simulink model "DiscretePiController"  (R2023a)
settings: Solver=VariableStepAuto  StartTime=0.0  StopTime=10.0  RelTol=1e-3
model workspace (MAT data in the model file):
  Ts = 0.1
  ki = 1
  kp = 0.2
settings Model: Creator=MY PC  LastModifiedBy=MY PC

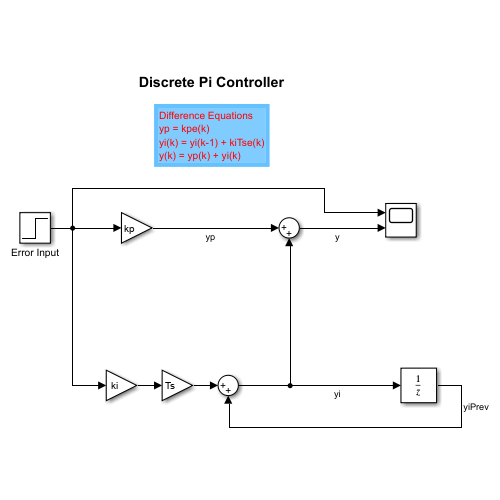
[thumbnail: Simulink's stored preview of the top-level diagram]
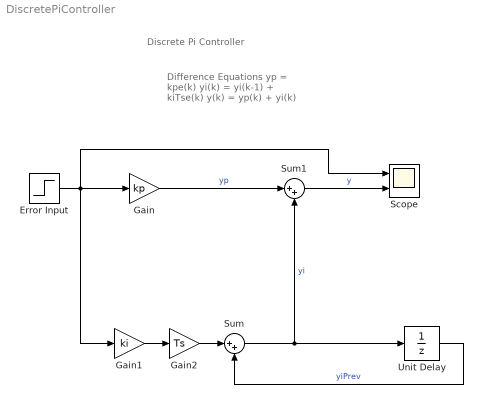
== system DiscretePiController ==
  note: Difference Equations
      | yp = kpe(k)
      | yi(k) = yi(k-1) + kiTse(k)
      | y(k) = yp(k) + yi(k)
  note: Discrete Pi Controller
  Error Input : Step  SampleTime=Ts
  Gain : Gain  Gain=kp
  Gain1 : Gain  Gain=ki
  Gain2 : Gain  Gain=Ts
  Scope : Scope  NumInputPorts=2
  Sum : Sum  Inputs=|++
  Sum1 : Sum  Inputs=|++
  Unit Delay : UnitDelay  SampleTime=Ts  HasFrameUpgradeWarning=on
  wires:
  Error Input/1 -> Scope/1, Gain/1, Gain1/1
  Gain/1 -> Sum1/1  "yp"
  Unit Delay/1 -> Sum/2  "yiPrev"
  Sum/1 -> Unit Delay/1, Sum1/2  "yi"
  Gain1/1 -> Gain2/1
  Gain2/1 -> Sum/1
  Sum1/1 -> Scope/2  "y"
